simulink library "INP_IMU_Comp"  (R2023b)
settings: Solver=VariableStepAuto  StartTime=0.0  StopTime=10.0  RelTol=1e-3
settings Model: Creator=blatak  LastModifiedBy=blatak
settings ModelReferenceCC: EnableRefExpFcnMdlSchedulingChecks=on

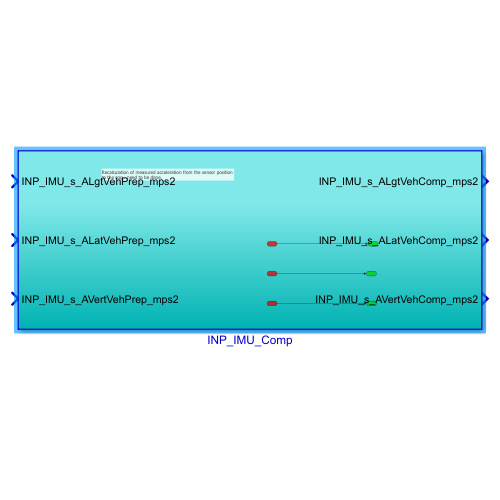
[thumbnail: Simulink's stored preview of the top-level diagram]
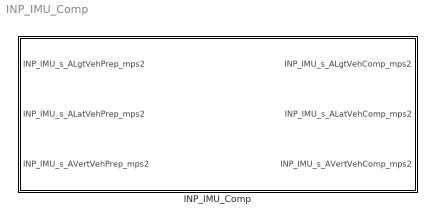
== system INP_IMU_Comp ==
  INP_IMU_Comp : Subsystem

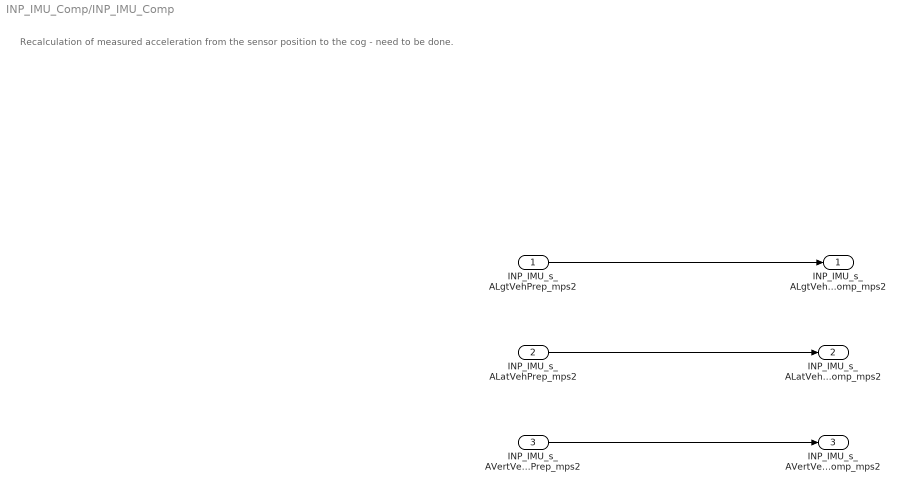
== system INP_IMU_Comp/INP_IMU_Comp ==
  note: Recalculation of measured acceleration from the sensor position to the cog - need to be done.
  INP_IMU_s_ALgtVehPrep_mps2 : Inport
  INP_IMU_s_ALatVehPrep_mps2 : Inport  Port=2
  INP_IMU_s_AVertVehPrep_mps2 : Inport  Port=3
  INP_IMU_s_ALgtVehComp_mps2 : Outport
  INP_IMU_s_ALatVehComp_mps2 : Outport  Port=2
  INP_IMU_s_AVertVehComp_mps2 : Outport  Port=3
  wires:
  INP_IMU_s_ALgtVehPrep_mps2/1 -> INP_IMU_s_ALgtVehComp_mps2/1
  INP_IMU_s_ALatVehPrep_mps2/1 -> INP_IMU_s_ALatVehComp_mps2/1
  INP_IMU_s_AVertVehPrep_mps2/1 -> INP_IMU_s_AVertVehComp_mps2/1
